simulink model "plMicrogridIslandOperation"  (Simulink 8.8)
settings: Solver=ode45  StartTime=0.0  StopTime=20  MaxStep=1e-3  RelTol=1e-6  EnableMultiTasking=on
undefined symbols (not defined in the file or in its folder): plecs
settings Model: SuppressorTable=22 serialization::archive 11 0 3 0 0 0 0 0  Creator=manaswini  LastModifiedBy=seananderson  ExtModeAutoUpdateStatusClock=off
settings OptimizationCC: ExpressionDepthLimit=2147483647
settings DebuggingCC: SaveWithParameterizedLinksMsg=none  MaxConsecutiveZCsMsg=none  SolverPrmCheckMsg=warning
settings HardwareCC: TargetHWDeviceType=32-bit Generic
settings GRTTargetCC: TargetFcnLib=ansi_tfl_tmw.mat  GeneratePreprocessorConditionals=Use local settings

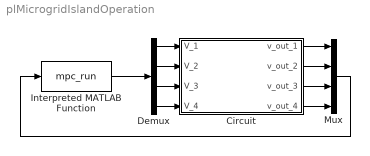
== system plMicrogridIslandOperation ==
  Circuit : Subsystem  LoadFcn=plecs('sl', 200);  InitFcn=plecs('sl', 214);  StartFcn=plecs('sl', 208);  StopFcn=plecs('sl', 209);  mask(PlecsCircuit){PLECSData=<binary blob, 38028 chars, not shown>}
      mask prompts: PLECSData "PLECS Data (Do not delete or modify!)"
      mask init:
      | % PLACE CUSTOM INITIALIZATIONS ABOVE
      | % DO NOT REMOVE
      | plecs('sl', 215);
      | % DO NOT REMOVE
      settings: CopyFcn=plecs('sl', 203);  DeleteFcn=plecs('sl', 205);  UndoDeleteFcn=plecs('sl', 206);  PreSaveFcn=plecs('sl', 211);  PostSaveFcn=plecs('sl', 201);  NameChangeFcn=plecs('sl', 210);  DestroyFcn=plecs('sl', 207);  PreCopyFcn=plecs('sl', 216);  OpenFcn=plecs('sl', 202);  ErrorFcn=plerrorfcn
      mask Help: web(['file:///' fullfile(plecsdoc, 'creatingacircuit.html')])
      mask Display: disp('PLECS\nCircuit')
  Demux : Demux
  Interpreted MATLAB Function : MATLABFcn  MATLABFcn=mpc_run
  Mux : Mux
  wires:
  Interpreted MATLAB Function/1 -> Demux/1
  Demux/1 -> Circuit/1(V_1)
  Demux/2 -> Circuit/2(V_2)
  Demux/3 -> Circuit/3(V_3)
  Demux/4 -> Circuit/4(V_4)
  Circuit/3(v_out_3) -> Mux/3
  Circuit/4(v_out_4) -> Mux/4
  Circuit/1(v_out_1) -> Mux/1
  Circuit/2(v_out_2) -> Mux/2
  Mux/1 -> Interpreted MATLAB Function/1

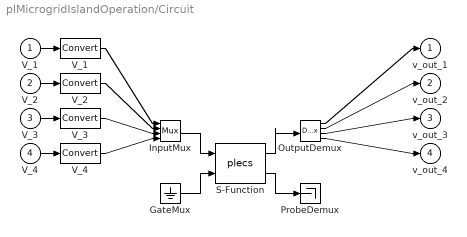
== system plMicrogridIslandOperation/Circuit ==
  V_1 : Inport  PortDimensions=1
  V_2 : Inport  Port=2  PortDimensions=1
  V_3 : Inport  Port=3  PortDimensions=1
  V_4 : Inport  Port=4  PortDimensions=1
  " GateMux " : Ground
  " InputMux " : Mux  Inputs=[ 1 1 1 1 ]
  " OutputDemux " : Demux  Outputs=[ 1 1 1 1 ]
  " ProbeDemux " : Terminator
  " S-Function " : S-Function  FunctionName=plecs  SFunctionDeploymentMode=off  EnableBusSupport=off
  " V_1 " : DataTypeConversion  SaturateOnIntegerOverflow=on  RndMeth=Zero
  " V_2 " : DataTypeConversion  SaturateOnIntegerOverflow=on  RndMeth=Zero
  " V_3 " : DataTypeConversion  SaturateOnIntegerOverflow=on  RndMeth=Zero
  " V_4 " : DataTypeConversion  SaturateOnIntegerOverflow=on  RndMeth=Zero
  v_out_1 : Outport  PortDimensions=1
  v_out_2 : Outport  Port=2  PortDimensions=1
  v_out_3 : Outport  Port=3  PortDimensions=1
  v_out_4 : Outport  Port=4  PortDimensions=1
  wires:
  " S-Function "/2 -> " ProbeDemux "/1
  " GateMux "/1 -> " S-Function "/2
  " InputMux "/1 -> " S-Function "/1
  " S-Function "/1 -> " OutputDemux "/1
  V_1/1 -> " V_1 "/1
  " V_1 "/1 -> " InputMux "/1
  V_2/1 -> " V_2 "/1
  " V_2 "/1 -> " InputMux "/2
  V_3/1 -> " V_3 "/1
  " V_3 "/1 -> " InputMux "/3
  V_4/1 -> " V_4 "/1
  " V_4 "/1 -> " InputMux "/4
  " OutputDemux "/1 -> v_out_1/1
  " OutputDemux "/2 -> v_out_2/1
  " OutputDemux "/3 -> v_out_3/1
  " OutputDemux "/4 -> v_out_4/1
